simulink model "ValveSim"  (R2021b)
settings: Solver=VariableStepAuto  StartTime=0.0  StopTime=10.0  RelTol=1e-3
libraries: nesl_utility x9, fl_lib x8, simulink x1, simulink_extras x1
settings Model: Creator=rasmu  LastModifiedBy=martin

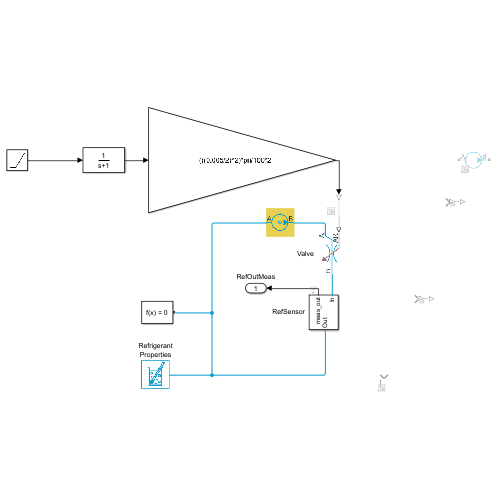
[thumbnail: Simulink's stored preview of the top-level diagram]
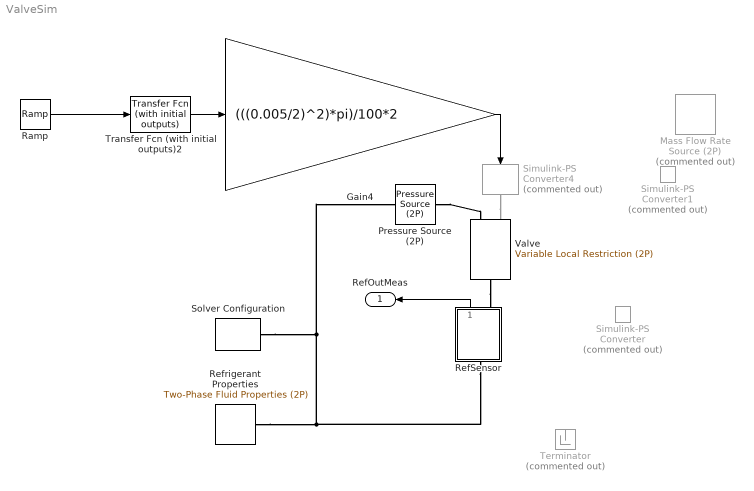
== system ValveSim ==
  Gain4 : Gain  Gain=(((0.005/2)^2)*pi)/100*2
  Mass Flow Rate Source (2P) : fl_lib/Two-Phase Fluid/Sources/Mass Flow Rate Source (2P)  Commented=on  power_spec=foundation.enum.power_spec.isentropic  mass_flow=0 kg/s  area_A=0.01 m^2  area_B=0.01 m^2
      settings: SourceProductBaseCode=SS  InternalSimscapePortConfiguration="{\"Bottom\":[],\"Left\":[{\"id\":\"A\",\"label\":\"A\",\"type\":\"foundation.two_phase_fluid.two_phase_fluid\"}],\"Right\":[{\"id\":\"B\",\"label\":\"B\",\"type\":\"foundation.two_phase_fluid.two_phase_fluid\"}],\"Top\":[]}"
  Pressure Source (2P) : fl_lib/Two-Phase Fluid/Sources/Pressure Source (2P)  power_spec=foundation.enum.power_spec.isentropic  pressure_differential=10 bar  area_A=0.01 m^2  area_B=0.01 m^2
      settings: SourceProductBaseCode=SS  InternalSimscapePortConfiguration="{\"Bottom\":[],\"Left\":[{\"id\":\"A\",\"label\":\"A\",\"type\":\"foundation.two_phase_fluid.two_phase_fluid\"}],\"Right\":[{\"id\":\"B\",\"label\":\"B\",\"type\":\"foundation.two_phase_fluid.two_phase_fluid\"}],\"Top\":[]}"
  Ramp : simulink/Sources/Ramp  slope=100/5000  start=0  InitialOutput=0
  RefSensor : Subsystem
      settings: PortSchema="{\"entries\":[{\"content\":{\"sides\":[{\"content\":{\"connectorIds\":[\"LConn1\",\"Out1\"]},\"type\":\"ConnectorPlacement.EquallySpacedRectSide\",\"uuid\":\"384ca129-c08e-4242-8b56-38a57a5275bd\"},{\"content\":{\"connectorIds\":[\"RConn1\"],\"side\":\"RIGHT\"},\"type\":\"ConnectorPlacement.EquallySpacedRectSide\",\"uuid\":\"d8d27130-51db-4533-93b1-df7418a29f3a\"},{\"content\":{\"connectorIds\":[],\"side\":\"TOP\"},\"type\":\"ConnectorPlacement.EquallySpacedRectSide\",\"uuid\":\"67192aad-d15e-443e-8c24-a3a889184c8d\"},{\"content\":{\"connectorIds\":[],\"side\":\"BOTTOM\"},\"type\":\"ConnectorPlacement.EquallySpacedRectSide\",\"uuid\":\"18e5bc3a-5c8d-47f7-9803-91861ffb04f2\"}]},\"type\":\"ConnectorPlacement.EquallySpacedConnector\",\"uuid\":\"971e7a76-7cfc-4fb4-bbb6-a40c097b0bda\"}],\"packageUris\":[\"http://schema.mathworks.com/mf0/Connector/19700101\"],\"version\":\"1.0\"}"
  Refrigerant Properties : fl_lib/Two-Phase Fluid/Utilities/Two-Phase Fluid Properties (2P)  u_min=RefrigerantPropertyTables.u_min kJ/kg  u_max=RefrigerantPropertyTables.u_max kJ/kg  p_TLU=RefrigerantPropertyTables.p MPa  p_crit=RefrigerantPropertyTables.p_crit MPa  critical_region=foundation.enum.critical_region.clip  p_crit_fraction=0.12  p_atm=0.101325 MPa  q_rev=0.01 Pa  unorm_liq=RefrigerantPropertyTables.liquid.unorm  v_liq=RefrigerantPropertyTables.liquid.v m^3/kg  s_liq=RefrigerantPropertyTables.liquid.s kJ/(K*kg)  T_liq=RefrigerantPropertyTables.liquid.T K  nu_liq=RefrigerantPropertyTables.liquid.nu mm^2/s  k_liq=RefrigerantPropertyTables.liquid.k W/(m*K)  Pr_liq=RefrigerantPropertyTables.liquid.Pr  u_sat_liq=RefrigerantPropertyTables.liquid.u_sat kJ/kg  unorm_vap=RefrigerantPropertyTables.vapor.unorm  v_vap=RefrigerantPropertyTables.vapor.v m^3/kg  s_vap=RefrigerantPropertyTables.vapor.s kJ/(K*kg)  T_vap=RefrigerantPropertyTables.vapor.T K  nu_vap=RefrigerantPropertyTables.vapor.nu mm^2/s  k_vap=RefrigerantPropertyTables.vapor.k W/(m*K)  Pr_vap=RefrigerantPropertyTables.vapor.Pr  u_sat_vap=RefrigerantPropertyTables.vapor.u_sat kJ/kg
      settings: SourceProductBaseCode=SS  InternalSimscapePortConfiguration="{\"Bottom\":[],\"Left\":[],\"Right\":[{\"id\":\"A\",\"label\":\"\",\"type\":\"foundation.two_phase_fluid.two_phase_fluid\"}],\"Top\":[]}"
  Simulink-PS Converter : nesl_utility/Simulink-PS Converter  Commented=on  PhysicalDomain=network_engine_domain  SubClassName=ps_input  LeftPortType=input  RightPortType=output  PseudoPeriodic=off  Frequencies=[]  NoiseDistribution=none  NoiseParameters=[]  Unit=1  AffineConversion=off  FilteringAndDerivatives=provide  SimscapeFilterOrder=1  InputFilterTimeConstant=0.001  UdotUserProvided=0
      settings: SourceProductBaseCode=PW,SS
  Simulink-PS Converter1 : nesl_utility/Simulink-PS Converter  Commented=on  PhysicalDomain=network_engine_domain  SubClassName=ps_input  LeftPortType=input  RightPortType=output  PseudoPeriodic=off  Frequencies=[]  NoiseDistribution=none  NoiseParameters=[]  Unit=1  AffineConversion=off  FilteringAndDerivatives=provide  SimscapeFilterOrder=1  InputFilterTimeConstant=0.001  UdotUserProvided=0
      settings: SourceProductBaseCode=PW,SS
  Simulink-PS Converter4 : nesl_utility/Simulink-PS Converter  Commented=on  PhysicalDomain=network_engine_domain  SubClassName=ps_input  LeftPortType=input  RightPortType=output  PseudoPeriodic=off  Frequencies=[]  NoiseDistribution=none  NoiseParameters=[]  Unit=m^2  AffineConversion=off  FilteringAndDerivatives=zero  SimscapeFilterOrder=1  InputFilterTimeConstant=0.001  UdotUserProvided=1
      settings: SourceProductBaseCode=PW,SS
  Solver Configuration : nesl_utility/Solver Configuration  PhysicalDomain=network_engine_domain  SubClassName=solver  LeftPortType=input  RightPortType=generic  Tones=[]  Harmonics=[]  SimulateNoise=off  Profile=off  UseLocalSampling=off  EnableSwitchedLinearOptims=on  FrequencyDomain=off  UseCCode=off  RelTol=0.001  AbsTol=1e-06  MinStep=1e-09  ToWorkspace=off  RevertToSquareIcSolve=off  NumHomotopyIterations=100  PhasorMode=off  PhasorModeNumHarmonics=1  DoDC=off  ResidualTolerance=1e-3  UseLocalSolver=off  LocalSolverChoice=NE_BACKWARD_EULER_ADVANCER  LocalSolverSampleTime=.01  DoFixedCost=off  MaxNonlinIter=3  MaxModeIter=2  ComputeImpulses=off  ImpulseIterations=2  LinearAlgebra=auto  EquationFormulation=NE_TIME_EF  DelaysMemoryBudget=1024  AutomaticFiltering=on  FilteringTimeConstant=0.001  PartitionStorageMethod=AS_NEEDED  PartitionMemoryBudget=1024  PartitionMethod=FAST
      settings: SourceProductBaseCode=PW,SS
  Terminator : Terminator  Commented=on
  Transfer Fcn (with initial outputs)2 : simulink_extras/Additional Linear/Transfer Fcn (with initial outputs)  N=[1]  D="[1  1]"  Y0=0  U0=0
  Valve : fl_lib/Two-Phase Fluid/Elements/Variable Local Restriction (2P)  min_area=10e-10 mm^2  max_area=100 mm^2  area=(20/2)^2*pi mm^2  Cd=0.64  B_lam=0.999
      settings: SourceProductBaseCode=SS  InternalSimscapePortConfiguration="{\"Bottom\":[],\"Left\":[{\"id\":\"A\",\"label\":\"A\",\"type\":\"foundation.two_phase_fluid.two_phase_fluid\"},{\"id\":\"area_in\",\"label\":\"AR\",\"type\":\"input\"}],\"Right\":[{\"id\":\"B\",\"label\":\"B\",\"type\":\"foundation.two_phase_fluid.two_phase_fluid\"}],\"Top\":[]}"
  RefOutMeas : Outport
  wires:
  Ramp/1 -> Transfer Fcn (with initial outputs)2/1
  Transfer Fcn (with initial outputs)2/1 -> Gain4/1
  Gain4/1 -> Simulink-PS Converter4/1
  RefSensor/1(meas_out) -> RefOutMeas/1
  connections:
  Valve/RConn1 -- RefSensor/LConn1
  Simulink-PS Converter4/RConn1 -- Valve/LConn2
  Pressure Source (2P)/RConn1 -- Valve/LConn1
  RefSensor/RConn1 -- Refrigerant Properties/RConn1 -- Solver Configuration/RConn1 -- Pressure Source (2P)/LConn1

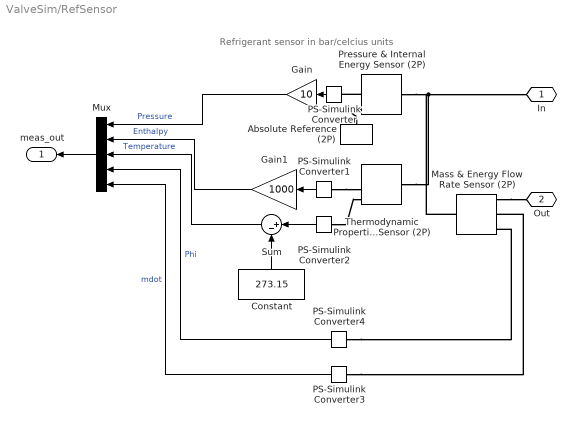
== system ValveSim/RefSensor ==
  note: Refrigerant sensor in bar/celcius units
  Absolute Reference (2P) : fl_lib/Two-Phase Fluid/Elements/Absolute Reference (2P)
      settings: SourceProductBaseCode=SS
  Constant : Constant  Value=273.15
  Gain : Gain  Gain=10
  Gain1 : Gain  Gain=1000
  Mass & Energy Flow Rate Sensor (2P) : fl_lib/Two-Phase Fluid/Sensors/Mass & Energy Flow Rate Sensor (2P)
      settings: SourceProductBaseCode=SS  InternalSimscapePortConfiguration="{\"Bottom\":[],\"Left\":[{\"id\":\"A\",\"label\":\"A\",\"type\":\"foundation.two_phase_fluid.two_phase_fluid\"}],\"Right\":[{\"id\":\"B\",\"label\":\"B\",\"type\":\"foundation.two_phase_fluid.two_phase_fluid\"},{\"id\":\"M\",\"label\":\"M\",\"type\":\"output\"},{\"id\":\"PHI\",\"label\":\"Phi\",\"type\":\"output\"}],\"Top\":[]}"
  Mux : Mux  Inputs=5
  PS-Simulink Converter{,1..4} (5 alike) : nesl_utility/PS-Simulink Converter  PhysicalDomain=network_engine_domain  SubClassName=ps_output  LeftPortType=input  RightPortType=output  PseudoPeriodic=off  Frequencies=[]  Unit=inherit  AffineConversion=off
      settings: SourceProductBaseCode=PW,SS
  Pressure & Internal Energy Sensor (2P) : fl_lib/Two-Phase Fluid/Sensors/Pressure & Internal Energy Sensor (2P)
      settings: SourceProductBaseCode=SS  InternalSimscapePortConfiguration="{\"Bottom\":[],\"Left\":[{\"id\":\"A\",\"label\":\"A\",\"type\":\"foundation.two_phase_fluid.two_phase_fluid\"}],\"Right\":[{\"id\":\"B\",\"label\":\"B\",\"type\":\"foundation.two_phase_fluid.two_phase_fluid\"},{\"id\":\"P\",\"label\":\"P\",\"type\":\"output\"},{\"id\":\"U\",\"label\":\"U\",\"type\":\"output\"}],\"Top\":[]}"
  Sum : Sum  Inputs=|+-
  Thermodynamic Properties Sensor (2P) : fl_lib/Two-Phase Fluid/Sensors/Thermodynamic Properties Sensor (2P)
      settings: SourceProductBaseCode=SS  InternalSimscapePortConfiguration="{\"Bottom\":[],\"Left\":[{\"id\":\"A\",\"label\":\"A\",\"type\":\"foundation.two_phase_fluid.two_phase_fluid\"}],\"Right\":[{\"id\":\"T\",\"label\":\"T\",\"type\":\"output\"},{\"id\":\"H\",\"label\":\"h\",\"type\":\"output\"},{\"id\":\"V\",\"label\":\"v\",\"type\":\"output\"},{\"id\":\"S\",\"label\":\"s\",\"type\":\"output\"}],\"Top\":[]}"
  In : PMIOPort  Side=Left
  Out : PMIOPort  Port=2  Side=Right
  meas_out : Outport
  wires:
  Sum/1 -> Mux/3  "Temperature"
  PS-Simulink Converter1/1 -> Gain1/1
  Gain/1 -> Mux/1  "Pressure"
  PS-Simulink Converter2/1 -> Sum/1
  Mux/1 -> meas_out/1
  PS-Simulink Converter/1 -> Gain/1
  Constant/1 -> Sum/2
  Gain1/1 -> Mux/2  "Enthalpy"
  PS-Simulink Converter4/1 -> Mux/4  "Phi"
  PS-Simulink Converter3/1 -> Mux/5  "mdot"
  connections:
  Pressure & Internal Energy Sensor (2P)/LConn1 -- In/RConn1 -- Thermodynamic Properties Sensor (2P)/LConn1 -- Mass & Energy Flow Rate Sensor (2P)/LConn1
  PS-Simulink Converter1/LConn1 -- Thermodynamic Properties Sensor (2P)/RConn2
  Pressure & Internal Energy Sensor (2P)/RConn1 -- Absolute Reference (2P)/LConn1
  Pressure & Internal Energy Sensor (2P)/RConn2 -- PS-Simulink Converter/LConn1
  PS-Simulink Converter2/LConn1 -- Thermodynamic Properties Sensor (2P)/RConn1
  Mass & Energy Flow Rate Sensor (2P)/RConn1 -- Out/RConn1
  PS-Simulink Converter4/LConn1 -- Mass & Energy Flow Rate Sensor (2P)/RConn3
  PS-Simulink Converter3/LConn1 -- Mass & Energy Flow Rate Sensor (2P)/RConn2
